simulink model "file1"  (R2025b)
settings: Solver=VariableStepAuto  StartTime=0.0  StopTime=1  RelTol=1e-3
InitFcn:
  | Voc=32.9;
  | Iscn=8.21;
  | k=1.38e-23;
  | NS=54;
  | Np=1;
  | Gn=1000;
  | Kv=-0.123;
  | K1=0.0032;
  | T=301;
  | Tn=300;
  | q=1.6e-19;
  | I0n=9.85e-8;
  | Eg=1.12;
  | Ign=8.214;
  | Rs=0.221;
  | Rp=414.5;
  | a=1.0;
undefined symbols (not defined in the file): G
libraries: spsSeriesRLCBranchLib x2, spsVoltageMeasurementLib x2, spsControlledCurrentSourceLib x1, spsControlledVoltageSourceLib x1, spsCurrentMeasurementLib x1, simulink x1, sps_lib x1
settings Model: Creator=sagnikdey  LastModifiedBy=hp

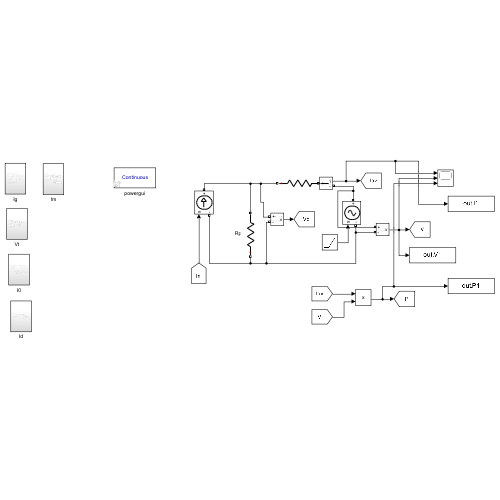
[thumbnail: Simulink's stored preview of the top-level diagram]
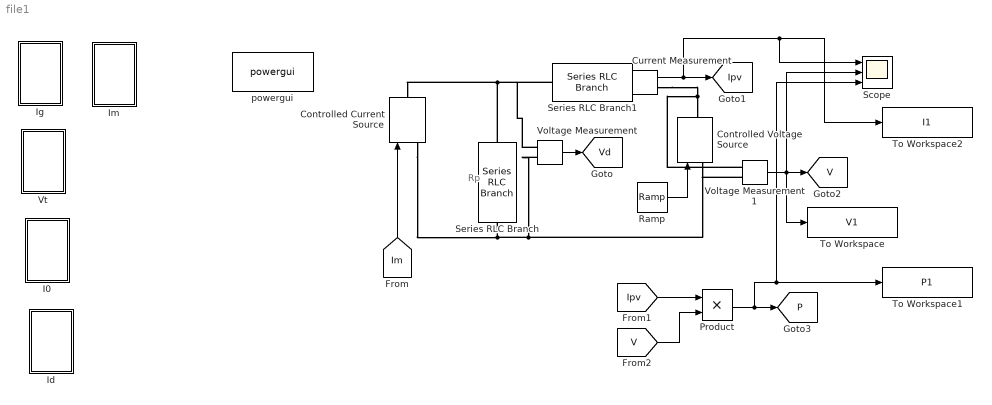
== system file1 ==
  note: Rp
  Controlled Current Source : spsControlledCurrentSourceLib/Controlled Current Source  Initialize=on  Source_Type=AC  Amplitude=0  Phase=0  Frequency=0  Measurements=None
  Controlled Voltage Source : spsControlledVoltageSourceLib/Controlled Voltage Source  Initialize=on  Source_Type=AC  Amplitude=0  Phase=0  Frequency=0  Measurements=None
  Current Measurement : spsCurrentMeasurementLib/Current Measurement  PhasorSimulation=off  OutputType=Complex  PSBequivalent=0
  I0 : Subsystem
  Id : Subsystem
  Ig : Subsystem
  Im : Subsystem
  Product : Product
  Ramp : simulink/Sources/Ramp  slope=32.9  start=0  InitialOutput=0
  Scope : Scope  NumInputPorts=3
      settings: ActiveDisplayYMinimum=-10.745882999165644  ActiveDisplayYMaximum=239.77779903095993
  Series RLC Branch : spsSeriesRLCBranchLib/Series RLC Branch  LConnTagsString=__new0  RConnTagsString=__new0  BranchType=R  Resistance=Rp  Inductance=1e-3  SetiL0=off  InitialCurrent=0  Capacitance=1e-6  Setx0=off  InitialVoltage=0  Measurements=None
  Series RLC Branch1 : spsSeriesRLCBranchLib/Series RLC Branch  LConnTagsString=__new0  RConnTagsString=__new0  BranchType=R  Resistance=Rs  Inductance=1e-3  SetiL0=off  InitialCurrent=0  Capacitance=1e-6  Setx0=off  InitialVoltage=0  Measurements=None
  To Workspace : ToWorkspace  VariableName=V1  SampleTime=-1
  To Workspace1 : ToWorkspace  VariableName=P1  SampleTime=-1
  To Workspace2 : ToWorkspace  VariableName=I1  SampleTime=-1
  Voltage Measurement : spsVoltageMeasurementLib/Voltage Measurement  PhasorSimulation=off  OutputType=Complex  PSBequivalent=0
  Voltage Measurement1 : spsVoltageMeasurementLib/Voltage Measurement  PhasorSimulation=off  OutputType=Complex  PSBequivalent=0
  Vt : Subsystem
  powergui : sps_lib/powergui  Priority=1  SimulationMode=Continuous  SampleTime=50e-6  frequency=60  Iterations=50  frequencyindice=0  Pbase=100e6  ErrMax=1e-4  UnitsV=kV  UnitsW=MW  buscounter=0  FunctionMessages=off  echomessages=off  EnableUseOfTLC=off  CurrentSourceSwitches=off  DisableSnubberDevices=off  DisableRonSwitches=off  DisableVfSwitches=off  DisplayEquations=off  AutomaticDiscreteSolvers=off  SolverType=Tustin/Backward Euler (TBE)  Interpol=off  ExternalGateDelay=off  methode=off  Ts=100  x0status=blocks  SPID=on  SwTol=0  HookPort=off  NonlinearTolerance=1e-4  nMaxIteration=100  ContinueOnMaxIteration=off  RestoreLinks=warning  ResistiveCurrentMeasurement=off  Frange=[0:2:500]  Ylog=off  Xlog=on  ShowGrid=off  save=off  variable=ZData  structure=0  ZoomFFT=off  StartTime=0.0  cycles=1  DisplayStyle=1  fundamental=60  FreqAxis=off  MaxFrequency=1000  frequencyindicesteady=1  RmsSteady=1  display=off
  tag scope: Ipv=global, P=global, V=global, Vd=global
  wires:
  [Im] -> Controlled Current Source/1
  Voltage Measurement/1 -> [Vd]
  Ramp/1 -> Controlled Voltage Source/1
  Current Measurement/1 -> To Workspace2/1, Scope/1, [Ipv]
  Voltage Measurement1/1 -> Scope/2, To Workspace/1, [V]
  [Ipv] -> Product/1
  [V] -> Product/2
  Product/1 -> Scope/3, To Workspace1/1, [P]
  connections:
  Series RLC Branch/RConn1 -- Voltage Measurement/LConn1 -- Series RLC Branch1/LConn1 -- Controlled Current Source/RConn1
  Controlled Current Source/LConn1 -- Voltage Measurement1/LConn2 -- Controlled Voltage Source/LConn1 -- Voltage Measurement/LConn2 -- Series RLC Branch/LConn1
  Current Measurement/LConn1 -- Series RLC Branch1/RConn1
  Current Measurement/RConn1 -- Voltage Measurement1/LConn1 -- Controlled Voltage Source/RConn1

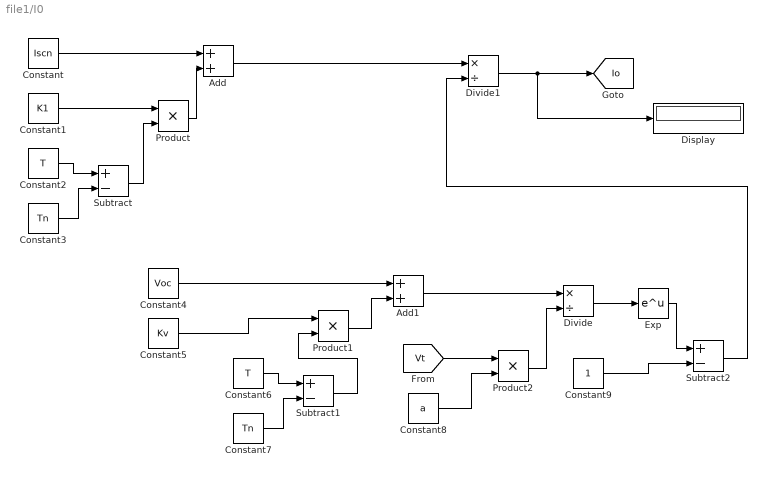
== system file1/I0 ==
  Add : Sum
  Add1 : Sum
  Constant : Constant  Value=Iscn
  Constant1 : Constant  Value=K1
  Constant2 : Constant  Value=T
  Constant3 : Constant  Value=Tn
  Constant4 : Constant  Value=Voc
  Constant5 : Constant  Value=Kv
  Constant6 : Constant  Value=T
  Constant7 : Constant  Value=Tn
  Constant8 : Constant  Value=a
  Constant9 : Constant
  Display : Display
  Divide : Product  Inputs=*/
  Divide1 : Product  Inputs=*/
  Exp : Math
  Product : Product
  Product1 : Product
  Product2 : Product
  Subtract : Sum  Inputs=+-
  Subtract1 : Sum  Inputs=+-
  Subtract2 : Sum  Inputs=+-
  tag scope: Io=global
  wires:
  Constant4/1 -> Add1/1
  Subtract1/1 -> Product1/2
  Constant1/1 -> Product/1
  Constant/1 -> Add/1
  Subtract2/1 -> Divide1/2
  [Vt] -> Product2/1
  Add/1 -> Divide1/1
  Product1/1 -> Add1/2
  Divide/1 -> Exp/1
  Divide1/1 -> Display/1, [Io]
  Constant7/1 -> Subtract1/2
  Product2/1 -> Divide/2
  Subtract/1 -> Product/2
  Constant2/1 -> Subtract/1
  Constant6/1 -> Subtract1/1
  Constant9/1 -> Subtract2/2
  Constant5/1 -> Product1/1
  Constant8/1 -> Product2/2
  Product/1 -> Add/2
  Constant3/1 -> Subtract/2
  Exp/1 -> Subtract2/1
  Add1/1 -> Divide/1

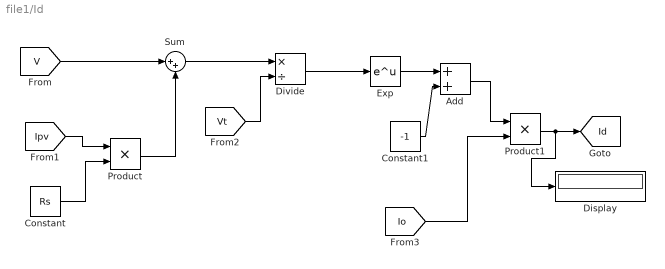
== system file1/Id ==
  Add : Sum
  Constant : Constant  Value=Rs
  Constant1 : Constant  Value=-1
  Display : Display
  Divide : Product  Inputs=*/
  Exp : Math
  Product : Product
  Product1 : Product
  Sum : Sum  Inputs=|++
  tag scope: Id=global
  wires:
  [Ipv] -> Product/1
  Product1/1 -> Display/1, [Id]
  [Io] -> Product1/2
  Sum/1 -> Divide/1
  [Vt] -> Divide/2
  Product/1 -> Sum/2
  Constant1/1 -> Add/2
  [V] -> Sum/1
  Exp/1 -> Add/1
  Constant/1 -> Product/2
  Add/1 -> Product1/1
  Divide/1 -> Exp/1

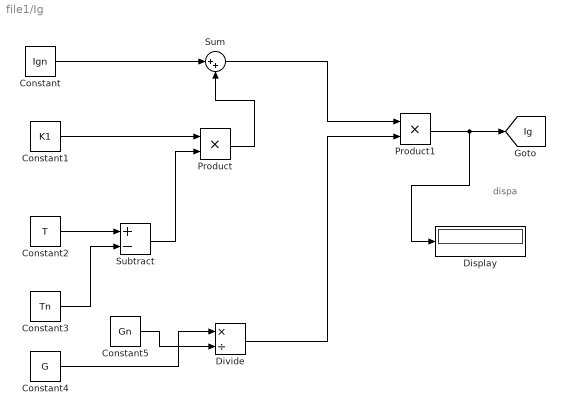
== system file1/Ig ==
  note: dispa
  Constant : Constant  Value=Ign
  Constant1 : Constant  Value=K1
  Constant2 : Constant  Value=T
  Constant3 : Constant  Value=Tn
  Constant4 : Constant  Value=G
  Constant5 : Constant  Value=Gn
  Display : Display
  Divide : Product  Inputs=*/
  Product : Product
  Product1 : Product
  Subtract : Sum  Inputs=+-
  Sum : Sum  Inputs=|++
  tag scope: Ig=global
  wires:
  Product/1 -> Sum/2
  Constant2/1 -> Subtract/1
  Constant/1 -> Sum/1
  Constant5/1 -> Divide/2
  Constant3/1 -> Subtract/2
  Divide/1 -> Product1/2
  Product1/1 -> Display/1, [Ig]
  Subtract/1 -> Product/2
  Sum/1 -> Product1/1
  Constant1/1 -> Product/1
  Constant4/1 -> Divide/1

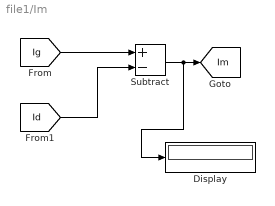
== system file1/Im ==
  Display : Display
  Subtract : Sum  Inputs=+-
  tag scope: Im=global
  wires:
  [Ig] -> Subtract/1
  [Id] -> Subtract/2
  Subtract/1 -> Display/1, [Im]

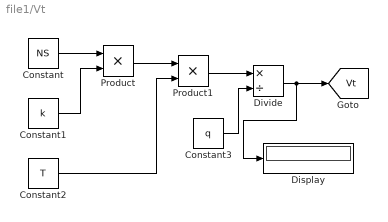
== system file1/Vt ==
  Constant : Constant  Value=NS
  Constant1 : Constant  Value=k
  Constant2 : Constant  Value=T
  Constant3 : Constant  Value=q
  Display : Display
  Divide : Product  Inputs=*/
  Product : Product
  Product1 : Product
  tag scope: Vt=global
  wires:
  Constant3/1 -> Divide/2
  Constant2/1 -> Product1/2
  Product1/1 -> Divide/1
  Product/1 -> Product1/1
  Constant/1 -> Product/1
  Constant1/1 -> Product/2
  Divide/1 -> Display/1, [Vt]
